simulink model "Reference_s"  (R2023a)
settings: Solver=VariableStepAuto  StartTime=0.0  StopTime=10.0  RelTol=1e-3
undefined symbols (not defined in the file): Tdref_ay_bp_ms2, Tdref_table, Tdref_v_bp_ms
settings Model: Creator=Tan_Tram  LastModifiedBy=Tan_Tram

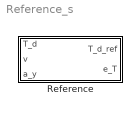
== system Reference_s ==
  Reference : Subsystem

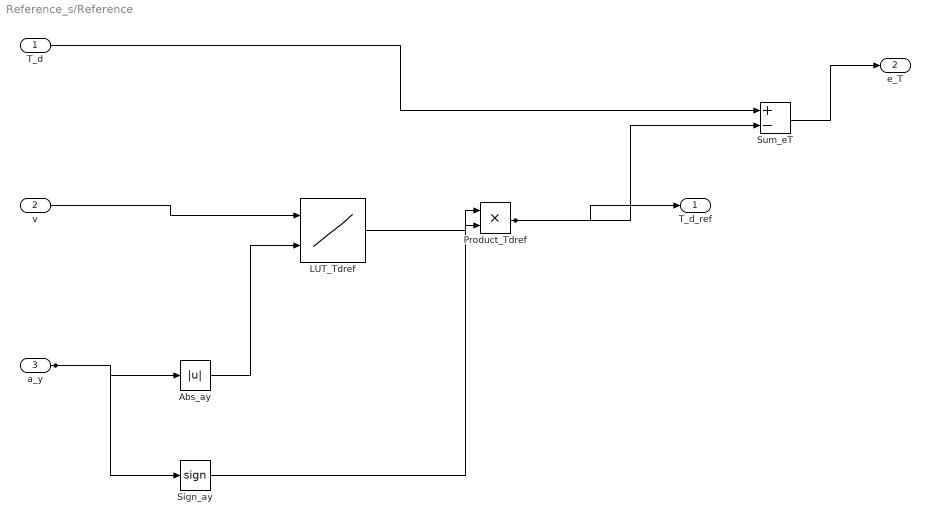
== system Reference_s/Reference ==
  T_d : Inport
  v : Inport  Port=2
  a_y : Inport  Port=3
  Abs_ay : Abs  SaturateOnIntegerOverflow=off
  LUT_Tdref : Lookup_n-D  BreakpointsForDimension1=Tdref_v_bp_ms  BreakpointsForDimension2=Tdref_ay_bp_ms2  Table=Tdref_table  ExtrapMethod=Clip  InternalRulePriority=Speed  RndMeth=Simplest
      settings: InputPortMap=u0,u1
  Product_Tdref : Product  Inputs=**
  Sign_ay : Signum
  Sum_eT : Sum  Inputs=+-
  T_d_ref : Outport
  e_T : Outport  Port=2
  wires:
  a_y/1 -> Abs_ay/1, Sign_ay/1
  v/1 -> LUT_Tdref/1
  Abs_ay/1 -> LUT_Tdref/2
  Sign_ay/1 -> Product_Tdref/1
  LUT_Tdref/1 -> Product_Tdref/2
  Product_Tdref/1 -> T_d_ref/1, Sum_eT/2
  T_d/1 -> Sum_eT/1
  Sum_eT/1 -> e_T/1
